simulink model "L2_T3_speed_inner_loop"  (R2026a)
settings: Solver=ode23tb  StartTime=0  StopTime=0.05  MaxStep=2e-05
settings Model: Creator=m  LastModifiedBy=m

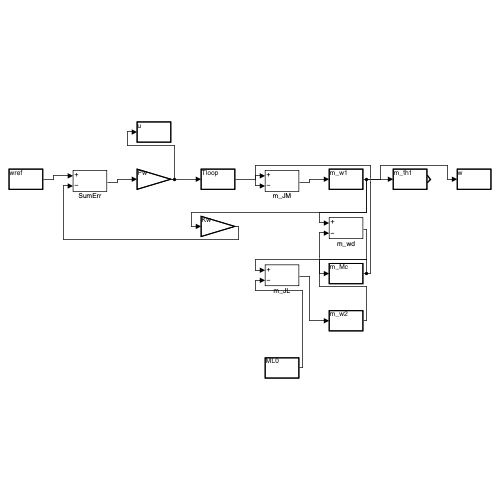
[thumbnail: Simulink's stored preview of the top-level diagram]
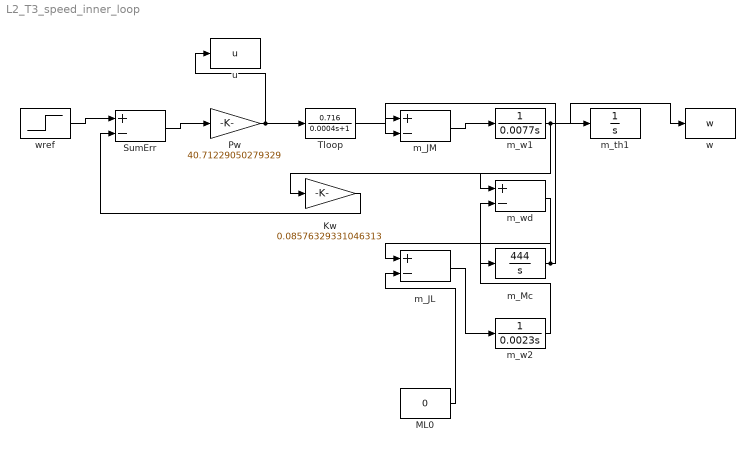
== system L2_T3_speed_inner_loop ==
  Kw : Gain  Gain=0.08576329331046313
  ML0 : Constant  Value=0
  Pw : Gain  Gain=40.71229050279329
  SumErr : Sum  Inputs=+-
  Tloop : TransferFcn  Numerator=0.716  Denominator=[0.0004 1]
  m_JL : Sum  Inputs=+-
  m_JM : Sum  Inputs=+-
  m_Mc : TransferFcn  Numerator=444  Denominator=[1 0]
  m_th1 : Integrator
  m_w1 : TransferFcn  Numerator=1  Denominator=[0.0077 0]
  m_w2 : TransferFcn  Numerator=1  Denominator=[0.0023 0]
  m_wd : Sum  Inputs=+-
  u : ToWorkspace  VariableName=u  SaveFormat=Structure With Time  SampleTime=-1
  w : ToWorkspace  VariableName=w  SaveFormat=Structure With Time  SampleTime=-1
  wref : Step  Time=0  FinalValue=8.977142857142857  SampleTime=0
  wires:
  m_JM/1 -> m_w1/1
  m_w1/1 -> m_wd/1, m_th1/1, Kw/1, w/1
  m_w2/1 -> m_wd/2
  m_wd/1 -> m_Mc/1
  m_Mc/1 -> m_JM/2, m_JL/1
  m_JL/1 -> m_w2/1
  wref/1 -> SumErr/1
  SumErr/1 -> Pw/1
  Pw/1 -> Tloop/1, u/1
  Tloop/1 -> m_JM/1
  ML0/1 -> m_JL/2
  Kw/1 -> SumErr/2
